simulink model "sldemo_varsize_multimodeFixSizeImpl"  (Simulink 7.6)
settings: Solver=FixedStepDiscrete  StartTime=0.0  StopTime=20  RelTol=1e-3
libraries: simulink x3
settings Model: Creator=The MathWorks Inc.
settings OptimizationCC: InitFltsAndDblsToZero=on
settings SFSimCC: SimParseCustomCode=off

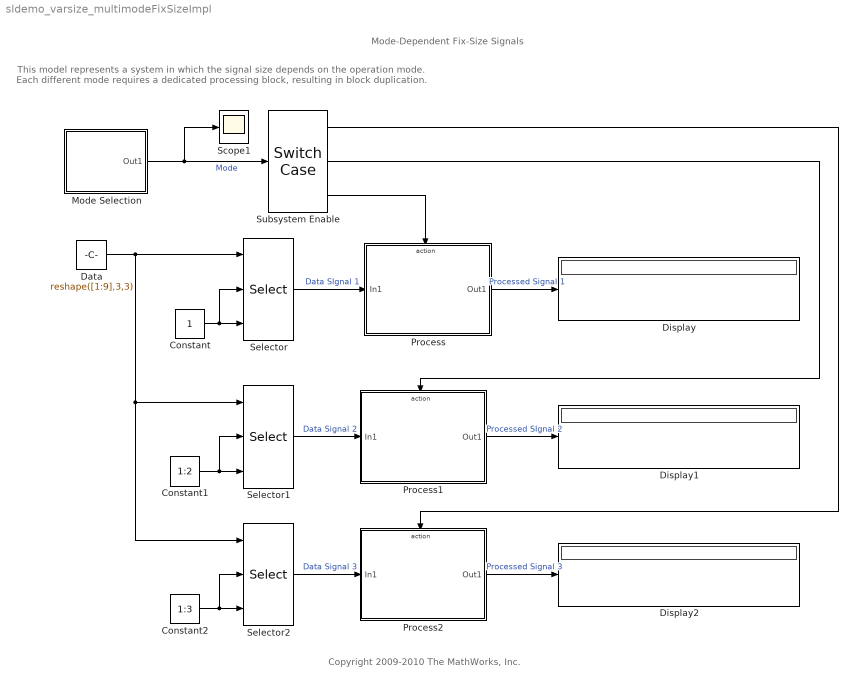
== system sldemo_varsize_multimodeFixSizeImpl ==
  note: Mode-Dependent Fix-Size Signals
  note: This model represents a system in which the signal size depends on the operation mode.
      | Each different mode requires a dedicated processing block, resulting in block duplication.
  note: Copyright 2009-2010 The MathWorks, Inc.
  Constant : Constant
  Constant1 : Constant  Value=1:2
  Constant2 : Constant  Value=1:3
  Data : Constant  Value=reshape([1:9],3,3)
  Display : Display
  Display1 : Display
  Display2 : Display
  Mode Selection : Subsystem
  Process : Subsystem  TreatAsAtomicUnit=on
  Process1 : Subsystem  TreatAsAtomicUnit=on
  Process2 : Subsystem  TreatAsAtomicUnit=on
  Scope1 : Scope
      settings: TimeRange=20  YMin=0.5  YMax=3.5
  Selector : Selector  NumberOfDimensions=2  InputPortWidth=3  IndexOptions=Index vector (port),Index vector (port)  Indices=1:8,1:8  OutputSizes=1,1
  Selector1 : Selector  NumberOfDimensions=2  InputPortWidth=3  IndexOptions=Index vector (port),Index vector (port)  Indices=1:4,1:4  OutputSizes=1,1
  Selector2 : Selector  NumberOfDimensions=2  InputPortWidth=3  IndexOptions=Index vector (port),Index vector (port)  Indices=1:4,1:4  OutputSizes=1,1
  "Subsystem Enable " : SwitchCase  CaseConditions={1, 2, 3}  ShowDefaultCase=off
  wires:
  Selector/1 -> Process/1(In1)  "Data SIgnal 1"
  Selector1/1 -> Process1/1(In1)  "Data Signal 2"
  Selector2/1 -> Process2/1(In1)  "Data Signal 3"
  Constant/1 -> Selector/2, Selector/3
  Constant1/1 -> Selector1/3, Selector1/2
  Mode Selection/1(Out1) -> "Subsystem Enable "/1, Scope1/1  "Mode"
  Data/1 -> Selector/1, Selector2/1, Selector1/1
  "Subsystem Enable "/3 -> Process/Action
  "Subsystem Enable "/2 -> Process1/Action
  "Subsystem Enable "/1 -> Process2/Action
  Process/1(Out1) -> Display/1  "Processed Signal 1"
  Process1/1(Out1) -> Display1/1  "Processed SIgnal 2"
  Process2/1(Out1) -> Display2/1  "Processed Signal 3"
  Constant2/1 -> Selector2/3, Selector2/2

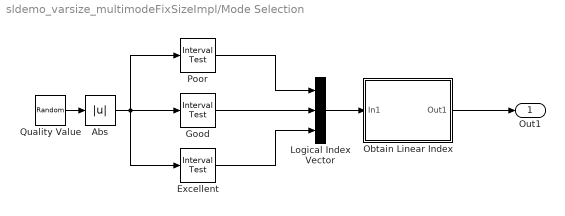
== system sldemo_varsize_multimodeFixSizeImpl/Mode Selection ==
  Abs : Abs
  Excellent : simulink/Logic and Bit Operations/Interval Test  SystemSampleTime=-1  IntervalClosedRight=off  uplimit=inf  IntervalClosedLeft=on  lowlimit=0.50  LogicOutDataTypeMode=uint8
  Good : simulink/Logic and Bit Operations/Interval Test  SystemSampleTime=-1  IntervalClosedRight=off  uplimit=0.50  IntervalClosedLeft=on  lowlimit=0.25  LogicOutDataTypeMode=uint8
  Logical Index Vector : Concatenate  NumInputs=3  Mode=Vector
  Obtain Linear Index : Subsystem
  Poor : simulink/Logic and Bit Operations/Interval Test  SystemSampleTime=-1  IntervalClosedRight=off  uplimit=0.25  IntervalClosedLeft=on  lowlimit=0.0  LogicOutDataTypeMode=uint8
  Quality Value : RandomNumber  Variance=.25  SampleTime=1
  Out1 : Outport
  wires:
  Obtain Linear Index/1(Out1) -> Out1/1
  Abs/1 -> Good/1, Poor/1, Excellent/1
  Good/1 -> Logical Index Vector/2
  Excellent/1 -> Logical Index Vector/3
  Poor/1 -> Logical Index Vector/1
  Logical Index Vector/1 -> Obtain Linear Index/1(In1)
  Quality Value/1 -> Abs/1

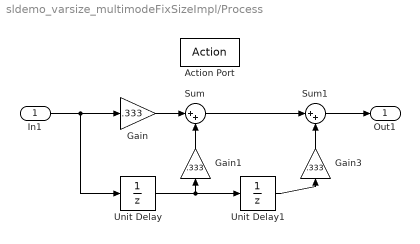
== system sldemo_varsize_multimodeFixSizeImpl/Process ==
  In1 : Inport
  Action Port : ActionPort  InitializeStates=reset  PropagateVarSize=During execution  ActionType=case
  Gain : Gain  Gain=.333
  Gain1 : Gain  Gain=.333
  Gain3 : Gain  Gain=.333
  Sum : Sum  Inputs=|++
  Sum1 : Sum  Inputs=|++
  Unit Delay : UnitDelay  SampleTime=-1
  Unit Delay1 : UnitDelay  SampleTime=-1
  Out1 : Outport  InitialOutput=[0]
  wires:
  Sum1/1 -> Out1/1
  Sum/1 -> Sum1/1
  Gain3/1 -> Sum1/2
  Unit Delay1/1 -> Gain3/1
  In1/1 -> Unit Delay/1, Gain/1
  Gain1/1 -> Sum/2
  Gain/1 -> Sum/1
  Unit Delay/1 -> Unit Delay1/1, Gain1/1

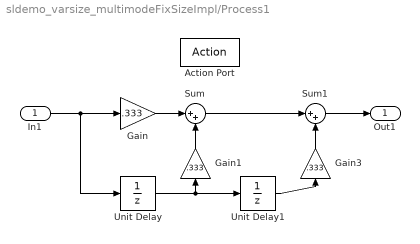
== system sldemo_varsize_multimodeFixSizeImpl/Process1 ==
  In1 : Inport
  Action Port : ActionPort  InitializeStates=reset  PropagateVarSize=During execution  ActionType=case
  Gain : Gain  Gain=.333
  Gain1 : Gain  Gain=.333
  Gain3 : Gain  Gain=.333
  Sum : Sum  Inputs=|++
  Sum1 : Sum  Inputs=|++
  Unit Delay : UnitDelay  SampleTime=-1
  Unit Delay1 : UnitDelay  SampleTime=-1
  Out1 : Outport  InitialOutput=[0]
  wires:
  Unit Delay/1 -> Gain1/1, Unit Delay1/1
  Gain/1 -> Sum/1
  Gain1/1 -> Sum/2
  In1/1 -> Gain/1, Unit Delay/1
  Unit Delay1/1 -> Gain3/1
  Gain3/1 -> Sum1/2
  Sum/1 -> Sum1/1
  Sum1/1 -> Out1/1

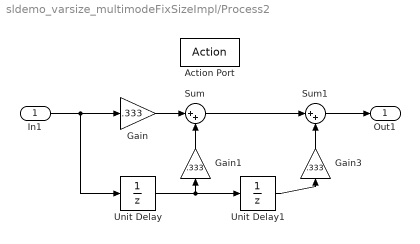
== system sldemo_varsize_multimodeFixSizeImpl/Process2 ==
  In1 : Inport
  Action Port : ActionPort  InitializeStates=reset  PropagateVarSize=During execution  ActionType=case
  Gain : Gain  Gain=.333
  Gain1 : Gain  Gain=.333
  Gain3 : Gain  Gain=.333
  Sum : Sum  Inputs=|++
  Sum1 : Sum  Inputs=|++
  Unit Delay : UnitDelay  SampleTime=-1
  Unit Delay1 : UnitDelay  SampleTime=-1
  Out1 : Outport  InitialOutput=[0]
  wires:
  Sum1/1 -> Out1/1
  Sum/1 -> Sum1/1
  Gain3/1 -> Sum1/2
  Unit Delay1/1 -> Gain3/1
  In1/1 -> Unit Delay/1, Gain/1
  Gain1/1 -> Sum/2
  Gain/1 -> Sum/1
  Unit Delay/1 -> Unit Delay1/1, Gain1/1

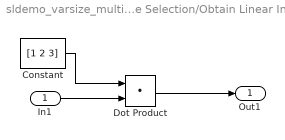
== system sldemo_varsize_multimodeFixSizeImpl/Mode Selection/Obtain Linear Index ==
  In1 : Inport
  Constant : Constant  Value=[1 2 3]
  Dot Product : DotProduct  OutDataTypeStr=Inherit: Inherit via internal rule
  Out1 : Outport
  wires:
  In1/1 -> Dot Product/2
  Dot Product/1 -> Out1/1
  Constant/1 -> Dot Product/1
